simulink model "findUnitVectors_th"  (R2018b)
settings: Solver=VariableStepAuto  StartTime=0.0  StopTime=0  RelTol=1e-3
libraries: findUnitVectors_ul x1
settings Model: Creator=MAE-NCSUCORE  LastModifiedBy=MAE-NCSUCORE

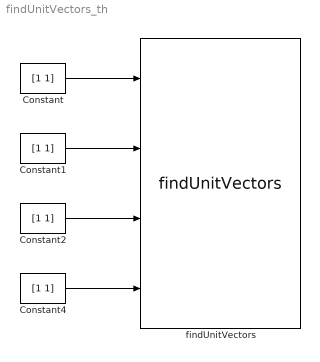
== system findUnitVectors_th ==
  Constant{,1..2,4} (4 alike) : Constant  Value=[1 1]
  findUnitVectors : findUnitVectors_ul/findUnitVectors  sideSeparation_cm=1.44  bottomASeparation_cm=1.43  bottomBSeparation_cm=2.75  cameraAngle_deg=45  sideEulerAngles=[0 180 180]  botEulerAngles=[0 90 -90]  slantEulerAngles=[0 135 180]
  wires:
  Constant4/1 -> findUnitVectors/4
  Constant2/1 -> findUnitVectors/3
  Constant1/1 -> findUnitVectors/2
  Constant/1 -> findUnitVectors/1
